simulink model "TwoTimeScale_ClosedLoop_Reference"  (R2023a)
settings: Solver=ode4  StartTime=0.0  StopTime=2  FixedStep=0.0005  RelTol=1e-3
settings Model: Creator=Fasih  LastModifiedBy=Fasih

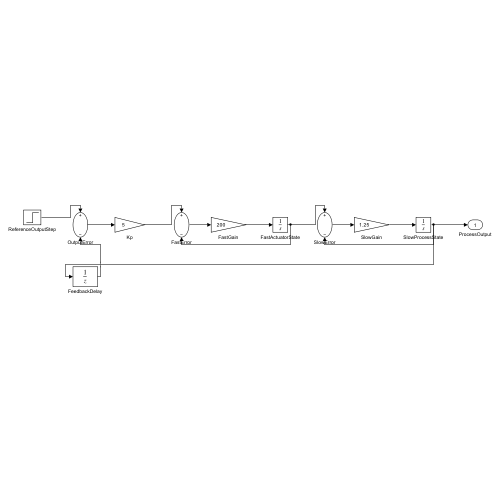
[thumbnail: Simulink's stored preview of the top-level diagram]
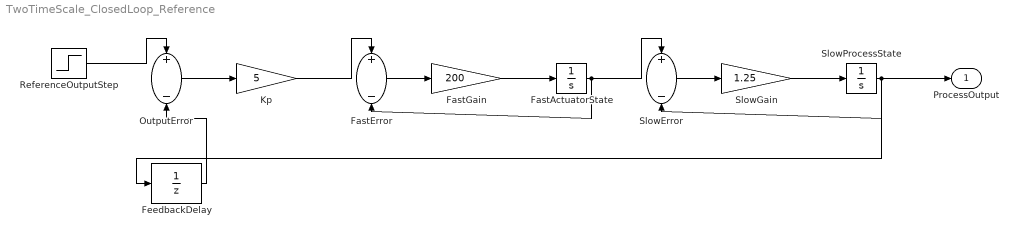
== system TwoTimeScale_ClosedLoop_Reference ==
  FastActuatorState : Integrator
  FastError : Sum  Inputs=+-
  FastGain : Gain  Gain=200
  FeedbackDelay : UnitDelay  SampleTime=0.0005  HasFrameUpgradeWarning=on
  Kp : Gain  Gain=5
  OutputError : Sum  Inputs=+-
  ReferenceOutputStep : Step  Time=0  SampleTime=0
  SlowError : Sum  Inputs=+-
  SlowGain : Gain  Gain=1.25
  SlowProcessState : Integrator
  ProcessOutput : Outport
  wires:
  ReferenceOutputStep/1 -> OutputError/1
  FeedbackDelay/1 -> OutputError/2
  OutputError/1 -> Kp/1
  Kp/1 -> FastError/1
  FastActuatorState/1 -> FastError/2, SlowError/1
  FastError/1 -> FastGain/1
  FastGain/1 -> FastActuatorState/1
  SlowProcessState/1 -> SlowError/2, ProcessOutput/1, FeedbackDelay/1
  SlowError/1 -> SlowGain/1
  SlowGain/1 -> SlowProcessState/1
